simulink model "SegwaySimulink"  (R2024a)
settings: Solver=VariableStepAuto  StartTime=0.0  StopTime=25  RelTol=1e-5
model workspace (MAT data in the model file):
  T = 0
values from neighbouring files (symbols this model uses):
  A = [0, 1, 0, 0; k5*k1/(k4*k1 - k2*k3), 0, 0, 0; 0, 0, 0, 1; - k2*k5/(k4*k1 - k2*k3), 0, 0, 0]    [linearizacija.m]
  B = [0; (-K*k1 - k3)/(k4*k1 - k2*k3); 0; 1/k1 + ((K*k1+k3)/(k4*k1-k2*k3))*(k2/k1)]    [linearizacija.m]
  C = [1, 0, 0, 0; 0, 1, 0, 0; 0, 0, 1, 0; 0, 0, 0, 1]    [linearizacija.m]
  PD_dteta = PDreg_acker(2)    [linearizacija.m]
  PD_dX = PDreg_acker(4)    [linearizacija.m]
  PD_teta = PDreg_acker(1)    [linearizacija.m]
  PD_x = PDreg_acker(3)    [linearizacija.m]
settings Model: NumberOfSteps=10  LastModifiedBy=Tamas
settings DebuggingCC: SignalInfNanChecking=error

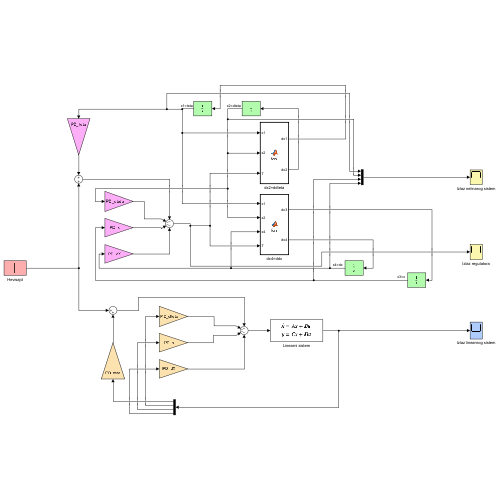
[thumbnail: Simulink's stored preview of the top-level diagram]
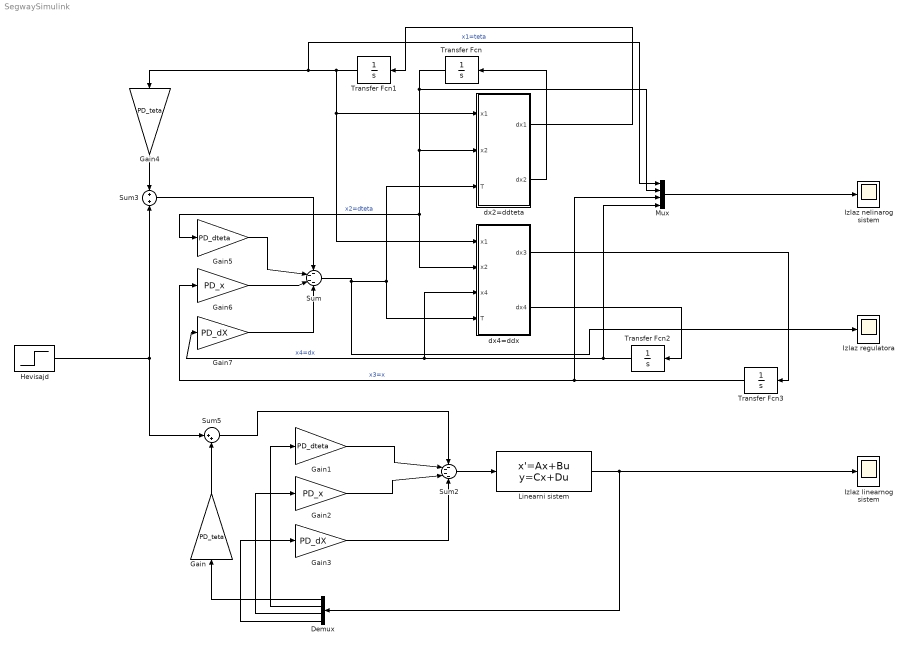
== system SegwaySimulink ==
  Demux : Demux
  Gain : Gain  Gain=PD_teta
  Gain1 : Gain  Gain=PD_dteta
  Gain2 : Gain  Gain=PD_x
  Gain3 : Gain  Gain=PD_dX
  Gain4 : Gain  Gain=PD_teta
  Gain5 : Gain  Gain=PD_dteta
  Gain6 : Gain  Gain=PD_x
  Gain7 : Gain  Gain=PD_dX
  Hevisajd : Step  After=pi/12  SampleTime=0
  Izlaz linearnog sistem : Scope
  Izlaz nelinarog sistem : Scope
  Izlaz regulatora : Scope
  Linearni sistem : StateSpace  A=A  B=B  C=C  D=[0;0;0;0]  InitialCondition=0
  Mux : Mux
  Sum : Sum  Inputs=----
  Sum2 : Sum  Inputs=----
  Sum3 : Sum  Inputs=+|+
  Sum5 : Sum  Inputs=|++
  Transfer Fcn{,1..3} (4 alike) : TransferFcn  Denominator=[1 0]
  dx2=ddteta : MATLAB Function  TreatAsAtomicUnit=on
  dx4=ddx : MATLAB Function  TreatAsAtomicUnit=on
  wires:
  dx2=ddteta/2(dx2) -> Transfer Fcn/1
  Transfer Fcn/1 -> dx4=ddx/2(x2), Gain5/1, dx2=ddteta/2(x2), Mux/2  "x2=dteta"
  Transfer Fcn1/1 -> dx4=ddx/1(x1), dx2=ddteta/1(x1), Mux/1, Gain4/1  "x1=teta"
  Linearni sistem/1 -> Demux/1, Izlaz linearnog sistem/1
  Hevisajd/1 -> Sum5/1, Sum3/2
  dx4=ddx/2(dx4) -> Transfer Fcn2/1
  Demux/1 -> Gain/1
  Sum2/1 -> Linearni sistem/1
  Demux/2 -> Gain1/1
  Demux/3 -> Gain2/1
  Demux/4 -> Gain3/1
  Sum5/1 -> Sum2/1
  Gain1/1 -> Sum2/2
  Gain2/1 -> Sum2/3
  Gain3/1 -> Sum2/4
  dx2=ddteta/1(dx1) -> Transfer Fcn1/1
  dx4=ddx/1(dx3) -> Transfer Fcn3/1
  Sum/1 -> Izlaz regulatora/1, dx4=ddx/4(T), dx2=ddteta/3(T)
  Gain7/1 -> Sum/4
  Gain6/1 -> Sum/3
  Gain5/1 -> Sum/2
  Sum3/1 -> Sum/1
  Transfer Fcn3/1 -> Mux/3, Gain6/1  "x3=x"
  Transfer Fcn2/1 -> Mux/4, dx4=ddx/3(x4), Gain7/1  "x4=dx"
  Mux/1 -> Izlaz nelinarog sistem/1
  Gain4/1 -> Sum3/1
  Gain/1 -> Sum5/2

== matlab function SegwaySimulink/dx2=ddteta ==
  data: dx1 output; x1 input; dx2 output; x2 input; T input
function [dx1,dx2] = fcn(x1, x2, T)
% x1 = theta
% x2 = d theta
% x3 = x
% x4 = d x
m = 85; % masa ručke
M = 3.5; % masa točkova
R = 0.1; % poluprečnik točkova
Iw = 0.1; % moment inercije točkova
Ir = 70; % moment inercije ručke
L = 1.7; % dužina ručke
g = 9.81;
%T = 0; % moment na točkovima
K = 1; 

%% kobasice

k1 = (M + m) * R + Iw/R;
k2 = m*L*R;
k3 = m*L;
k4 = Ir + m*L*L;
k5 = m*L*g;
k6 = m*L*R;

dx2 = ((T + k6*sin(x1) * x2 * x2 -    (k1  * k5 * sin(x1)  - K * T * k1)   /  (k3*cos(x1))) /(k2*cos(x1) - (k1*k4)/(k3*cos(x1))));
dx1= x2;

== matlab function SegwaySimulink/dx4=ddx ==
  data: dx3 output; x1 input; dx4 output; x2 input; x4 input; T input
function [dx3,dx4] = fcn(x1, x2, x4, T)
% x1 = theta
% x2 = d theta
% x3 = x
% x4 = d x
m = 85; % masa ručke
M = 3.5; % masa točkova
R = 0.1; % poluprečnik točkova
Iw = 0.1; % moment inercije točkova
Ir = 70; % moment inercije ručke
L = 1.7; % dužina ručke
g = 9.81;
%T = 0; % moment na točkovima
K = 1; 

% kobasice

k1 = (M + m) * R + Iw/R;
k2 = m*L*R;
k3 = m*L;
k4 = Ir + m*L*L;
k5 = m*L*g;
k6 = m*L*R;

dx4 = ((k5*sin(x1) - K*T - k4 *  ((T + k6 * sin(x1) * x2 * x2 -    (k1 * k5 * sin(x1)  - K * T * k1)   /  (k3*cos(x1))) /(k2*cos(x1) - k1*k4/(k3*cos(x1)))))/(k3*cos(x1)));
dx3=x4;
